simulink model "lacher"  (R2021b)
settings: Solver=VariableStepAuto  StartTime=0.0  StopTime=10  RelTol=1e-3
InitFcn:
  | Rm=3.15;
  | Lm=0.0015;
  | K=1.028;
  | fm=0.16805;
  | A2=0.0033153;
  | A1=0.045721;
  | L01=0.2625;
  | m2=0.24355;
  | A1tilde=A1+A2+m2*L01*L01;
  | A2tilde=A1tilde-A2;
  | f=0.070633;
  | lg1=0.16655703376925832;
  | m1=0.66984;
  | g=9.8;
  | Ceq=L01*m2*g+lg1*m1*g;
settings Model: PauseTimes=1  Creator=mimom  LastModifiedBy=dviol
settings DebuggingCC: UnconnectedInputMsg=none  UnconnectedOutputMsg=none  UnconnectedLineMsg=none
settings ModelReferenceCC: EnableRefExpFcnMdlSchedulingChecks=off
settings RTWCC: DLArmComputeVersion=20.02.1

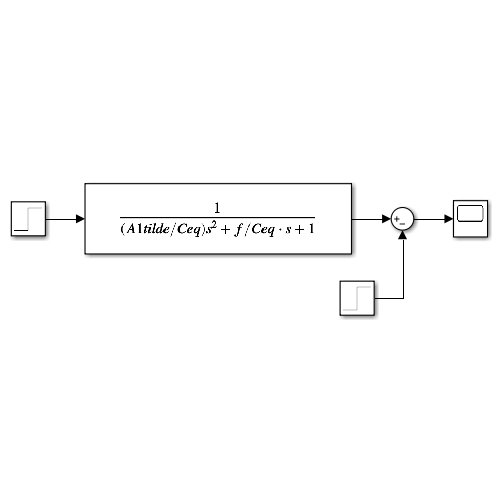
[thumbnail: Simulink's stored preview of the top-level diagram]
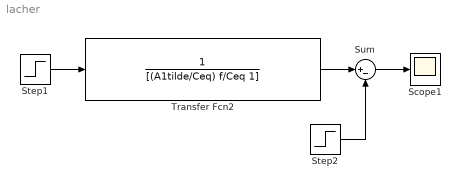
== system lacher ==
  Scope1 : Scope
  Step1 : Step  Time=0  After=pi/3  SampleTime=0
  Step2 : Step  Time=0  After=pi/3  SampleTime=0
  Sum : Sum  Inputs=|+-
  Transfer Fcn2 : TransferFcn  Denominator=[(A1tilde/Ceq) f/Ceq 1]
  wires:
  Step1/1 -> Transfer Fcn2/1
  Transfer Fcn2/1 -> Sum/1
  Sum/1 -> Scope1/1
  Step2/1 -> Sum/2
